simulink model "TD3_SimuAM"  (R2021b)
settings: Solver=ode45  StartTime=0.0  StopTime=8  RelTol=1e-3  EnableMultiTasking=on
values from neighbouring files (symbols this model uses):
  nu0 = 1    [TD3_SimuAM_Filtre.m]
  num = 10    [TD3_SimuAM_Filtre.m]
undefined symbols (not defined in the file or in its folder): A, B, nu1
settings Model: Creator=gscorlet  LastModifiedBy=Corentin
settings SolverCC: AlgebraicLoopSolver=TrustRegion
settings DataIOCC: LimitDataPoints=on  SaveFormat=Array  SignalLoggingSaveFormat=ModelDataLogs  ReturnWorkspaceOutputs=off  Refine=10
settings OptimizationCC: ExpressionDepthLimit=2147483647  InitFltsAndDblsToZero=on  LifeSpan=inf
settings DebuggingCC: SaveWithParameterizedLinksMsg=none  UnderspecifiedInitializationDetection=Classic  MergeDetectMultiDrivingBlocksExec=none  SignalResolutionControl=TryResolveAllWithWarning  SolverPrmCheckMsg=warning  MultiTaskDSMMsg=warning  MultiTaskCondExecSysMsg=none  FcnCallInpInsideContextMsg=warning  StateNameClashWarn=warning  SFUnexpectedBacktrackingDiag=warning  SFNoUnconditionalDefaultTransitionDiag=warning  SFExecutionAtInitializationDiag=none  SFMachineParentedDataDiag=warning  ArithmeticOperatorsInVariantConditions=warning
settings HardwareCC: ProdBitPerPointer=32  ProdBitPerSizeT=32  ProdBitPerPtrDiffT=32  ProdLargestAtomicFloat=None  ProdIntDivRoundTo=Undefined  ProdEndianess=Unspecified  ProdWordSize=32  ProdHWDeviceType=32-bit Generic
settings ModelReferenceCC: PropagateSignalLabelsOutOfModel=off
settings SFSimCC: SimUseLocalCustomCode=off  CustomCodeUndefinedFunction=UseInterfaceOnly
settings RTWCC: RTWUseLocalCustomCode=off
settings CodeAppCC: StateflowObjectComments=on
settings GRTTargetCC: TargetFcnLib=ansi_tfl_tmw.mat  TargetLangStandard=C89/C90 (ANSI)  CombineOutputUpdateFcns=off  GRTInterface=on
settings ConfigComp: CovMetricSettings=dw  CovSaveCumulativeToWorkspaceVar=on  CovSaveSingleToWorkspaceVar=on  CovExternalEMLEnable=off

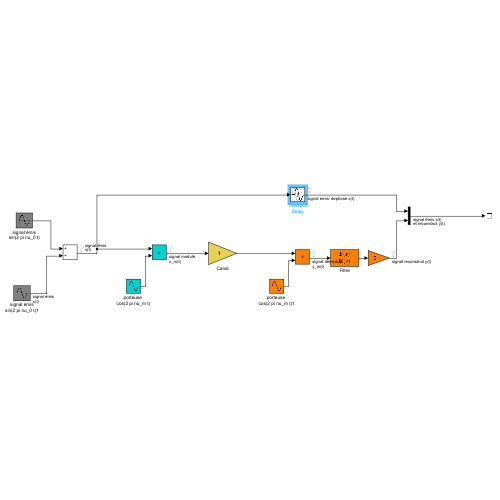
[thumbnail: Simulink's stored preview of the top-level diagram]
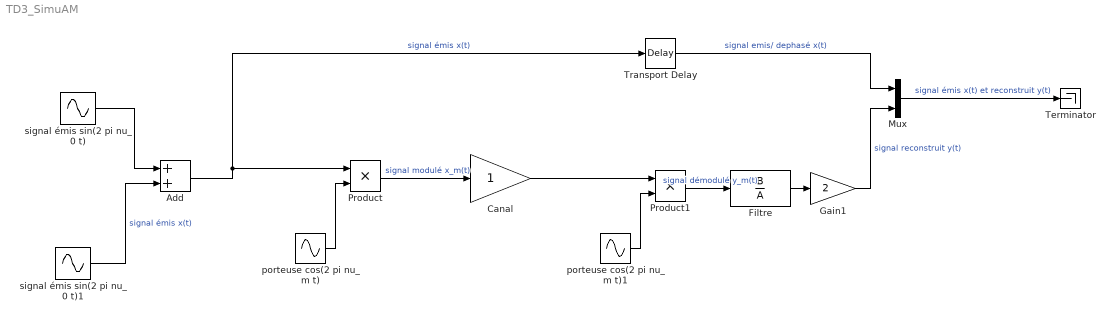
== system TD3_SimuAM ==
  Add : Sum
  Canal : Gain
  Filtre : TransferFcn  Numerator=B  Denominator=A
  Gain1 : Gain  Gain=2
  Mux : Mux  Inputs=2
  Product : Product  RndMeth=Zero
  Product1 : Product  RndMeth=Zero
  Terminator : Terminator
  Transport Delay : TransportDelay  DelayTime=0.66
  porteuse cos(2 pi nu_m t) : Sin  Frequency=2*pi*num  SampleTime=0
  porteuse cos(2 pi nu_m t)1 : Sin  Frequency=2*pi*num  SampleTime=0
  signal émis sin(2 pi nu_0 t) : Sin  Frequency=2*pi*nu0  SampleTime=0
  signal émis sin(2 pi nu_0 t)1 : Sin  Frequency=2*pi*nu1  SampleTime=0
  wires:
  porteuse cos(2 pi nu_m t)/1 -> Product/2
  Product/1 -> Canal/1  "signal modulé x_m(t)"
  Canal/1 -> Product1/1
  Product1/1 -> Filtre/1  "signal démodulé y_m(t)"
  Filtre/1 -> Gain1/1
  porteuse cos(2 pi nu_m t)1/1 -> Product1/2
  Gain1/1 -> Mux/2  "signal reconstruit y(t)"
  Transport Delay/1 -> Mux/1  "signal emis/ dephasé x(t)"
  Mux/1 -> Terminator/1  "signal émis x(t) et reconstruit y(t)"
  Add/1 -> Transport Delay/1, Product/1  "signal émis x(t)"
  signal émis sin(2 pi nu_0 t)/1 -> Add/1
  signal émis sin(2 pi nu_0 t)1/1 -> Add/2  "signal émis x(t)"
